simulink model "Model"  (R2020b)
settings: Solver=FixedStepDiscrete  StartTime=0.0  StopTime=inf  RelTol=1e-3
undefined symbols (not defined in the file): C12, designMultirateFIR, dt0
libraries: dspmlti4 x96, dspsrcs4 x89
(part 2 of 6)

== system Model/CORE_3_1/Path8 ==
  <IQ> : Inport
  Complex to Real-Imag : ComplexToRealImag
  Complex to Real-Imag1 : ComplexToRealImag
  Constant : Constant  Value=C12  SampleTime=dt0
  DDS_Gen1 : Subsystem
  FIR Dec1 : dspmlti4/FIR Decimation  FilterSource=Input port  h=designMultirateFIR(1,2)  D=2  filtStruct=Direct form  FilterObject=FDECIM  framing=Allow multirate processing  inputOffset=0  outputBufInitCond=0  roundingMode=Floor  overflowMode=off  firstCoeffDataTypeStr=Inherit: Same word length as input  firstCoeffMin=[]  firstCoeffMax=[]  firstCoeffLastDataTypeStr=Inherit: Same word length as input  outputDataTypeStr=Inherit: Same as accumulator  outputMin=[]  outputMax=[]  outputLastDataTypeStr=Inherit: Same as accumulator
  Freq1 : Constant  Value=2.4e6
  Mixer1 : Subsystem
  Real-Imag to Complex : RealImagToComplex
  Out1 : Outport
  wires:
  Constant/1 -> FIR Dec1/2
  Complex to Real-Imag/1 -> Mixer1/1(Input_I)
  Complex to Real-Imag1/1 -> Mixer1/3(DDS_I)
  Mixer1/2(Output_Q) -> Real-Imag to Complex/2
  Freq1/1 -> DDS_Gen1/1(In1)
  Complex to Real-Imag/2 -> Mixer1/2(Input_Q)
  Complex to Real-Imag1/2 -> Mixer1/4(DDS_Q)
  DDS_Gen1/1(Out1) -> Complex to Real-Imag1/1
  Real-Imag to Complex/1 -> FIR Dec1/1
  Mixer1/1(Output_I) -> Real-Imag to Complex/1
  FIR Dec1/1 -> Out1/1
  <IQ>/1 -> Complex to Real-Imag/1

== system Model/CORE_3_10/Path1 ==
  <IQ> : Inport
  Complex to Real-Imag : ComplexToRealImag
  Complex to Real-Imag1 : ComplexToRealImag
  Constant : Constant  Value=C12  SampleTime=dt0
  DDS_Gen1 : Subsystem
  FIR Dec1 : dspmlti4/FIR Decimation  FilterSource=Input port  h=designMultirateFIR(1,2)  D=2  filtStruct=Direct form  FilterObject=FDECIM  framing=Allow multirate processing  inputOffset=0  outputBufInitCond=0  roundingMode=Floor  overflowMode=off  firstCoeffDataTypeStr=Inherit: Same word length as input  firstCoeffMin=[]  firstCoeffMax=[]  firstCoeffLastDataTypeStr=Inherit: Same word length as input  outputDataTypeStr=Inherit: Same as accumulator  outputMin=[]  outputMax=[]  outputLastDataTypeStr=Inherit: Same as accumulator
  Freq1 : Constant  Value=2.4e6
  Mixer1 : Subsystem
  Real-Imag to Complex : RealImagToComplex
  Out1 : Outport
  wires:
  Constant/1 -> FIR Dec1/2
  Complex to Real-Imag/1 -> Mixer1/1(Input_I)
  Complex to Real-Imag1/1 -> Mixer1/3(DDS_I)
  Mixer1/2(Output_Q) -> Real-Imag to Complex/2
  Freq1/1 -> DDS_Gen1/1(In1)
  Complex to Real-Imag/2 -> Mixer1/2(Input_Q)
  Complex to Real-Imag1/2 -> Mixer1/4(DDS_Q)
  DDS_Gen1/1(Out1) -> Complex to Real-Imag1/1
  Real-Imag to Complex/1 -> FIR Dec1/1
  Mixer1/1(Output_I) -> Real-Imag to Complex/1
  FIR Dec1/1 -> Out1/1
  <IQ>/1 -> Complex to Real-Imag/1

== system Model/CORE_3_10/Path2 ==
  <IQ> : Inport
  Complex to Real-Imag : ComplexToRealImag
  Complex to Real-Imag1 : ComplexToRealImag
  Constant : Constant  Value=C12  SampleTime=dt0
  DDS_Gen1 : Subsystem
  FIR Dec1 : dspmlti4/FIR Decimation  FilterSource=Input port  h=designMultirateFIR(1,2)  D=2  filtStruct=Direct form  FilterObject=FDECIM  framing=Allow multirate processing  inputOffset=0  outputBufInitCond=0  roundingMode=Floor  overflowMode=off  firstCoeffDataTypeStr=Inherit: Same word length as input  firstCoeffMin=[]  firstCoeffMax=[]  firstCoeffLastDataTypeStr=Inherit: Same word length as input  outputDataTypeStr=Inherit: Same as accumulator  outputMin=[]  outputMax=[]  outputLastDataTypeStr=Inherit: Same as accumulator
  Freq1 : Constant  Value=2.4e6
  Mixer1 : Subsystem
  Real-Imag to Complex : RealImagToComplex
  Out1 : Outport
  wires:
  Constant/1 -> FIR Dec1/2
  Complex to Real-Imag/1 -> Mixer1/1(Input_I)
  Complex to Real-Imag1/1 -> Mixer1/3(DDS_I)
  Mixer1/2(Output_Q) -> Real-Imag to Complex/2
  Freq1/1 -> DDS_Gen1/1(In1)
  Complex to Real-Imag/2 -> Mixer1/2(Input_Q)
  Complex to Real-Imag1/2 -> Mixer1/4(DDS_Q)
  DDS_Gen1/1(Out1) -> Complex to Real-Imag1/1
  Real-Imag to Complex/1 -> FIR Dec1/1
  Mixer1/1(Output_I) -> Real-Imag to Complex/1
  FIR Dec1/1 -> Out1/1
  <IQ>/1 -> Complex to Real-Imag/1

== system Model/CORE_3_10/Path3 ==
  <IQ> : Inport
  Complex to Real-Imag : ComplexToRealImag
  Complex to Real-Imag1 : ComplexToRealImag
  Constant : Constant  Value=C12  SampleTime=dt0
  DDS_Gen1 : Subsystem
  FIR Dec1 : dspmlti4/FIR Decimation  FilterSource=Input port  h=designMultirateFIR(1,2)  D=2  filtStruct=Direct form  FilterObject=FDECIM  framing=Allow multirate processing  inputOffset=0  outputBufInitCond=0  roundingMode=Floor  overflowMode=off  firstCoeffDataTypeStr=Inherit: Same word length as input  firstCoeffMin=[]  firstCoeffMax=[]  firstCoeffLastDataTypeStr=Inherit: Same word length as input  outputDataTypeStr=Inherit: Same as accumulator  outputMin=[]  outputMax=[]  outputLastDataTypeStr=Inherit: Same as accumulator
  Freq1 : Constant  Value=2.4e6
  Mixer1 : Subsystem
  Real-Imag to Complex : RealImagToComplex
  Out1 : Outport
  wires:
  Constant/1 -> FIR Dec1/2
  Complex to Real-Imag/1 -> Mixer1/1(Input_I)
  Complex to Real-Imag1/1 -> Mixer1/3(DDS_I)
  Mixer1/2(Output_Q) -> Real-Imag to Complex/2
  Freq1/1 -> DDS_Gen1/1(In1)
  Complex to Real-Imag/2 -> Mixer1/2(Input_Q)
  Complex to Real-Imag1/2 -> Mixer1/4(DDS_Q)
  DDS_Gen1/1(Out1) -> Complex to Real-Imag1/1
  Real-Imag to Complex/1 -> FIR Dec1/1
  Mixer1/1(Output_I) -> Real-Imag to Complex/1
  FIR Dec1/1 -> Out1/1
  <IQ>/1 -> Complex to Real-Imag/1

== system Model/CORE_3_10/Path4 ==
  <IQ> : Inport
  Complex to Real-Imag : ComplexToRealImag
  Complex to Real-Imag1 : ComplexToRealImag
  Constant : Constant  Value=C12  SampleTime=dt0
  DDS_Gen1 : Subsystem
  FIR Dec1 : dspmlti4/FIR Decimation  FilterSource=Input port  h=designMultirateFIR(1,2)  D=2  filtStruct=Direct form  FilterObject=FDECIM  framing=Allow multirate processing  inputOffset=0  outputBufInitCond=0  roundingMode=Floor  overflowMode=off  firstCoeffDataTypeStr=Inherit: Same word length as input  firstCoeffMin=[]  firstCoeffMax=[]  firstCoeffLastDataTypeStr=Inherit: Same word length as input  outputDataTypeStr=Inherit: Same as accumulator  outputMin=[]  outputMax=[]  outputLastDataTypeStr=Inherit: Same as accumulator
  Freq1 : Constant  Value=2.4e6
  Mixer1 : Subsystem
  Real-Imag to Complex : RealImagToComplex
  Out1 : Outport
  wires:
  Constant/1 -> FIR Dec1/2
  Complex to Real-Imag/1 -> Mixer1/1(Input_I)
  Complex to Real-Imag1/1 -> Mixer1/3(DDS_I)
  Mixer1/2(Output_Q) -> Real-Imag to Complex/2
  Freq1/1 -> DDS_Gen1/1(In1)
  Complex to Real-Imag/2 -> Mixer1/2(Input_Q)
  Complex to Real-Imag1/2 -> Mixer1/4(DDS_Q)
  DDS_Gen1/1(Out1) -> Complex to Real-Imag1/1
  Real-Imag to Complex/1 -> FIR Dec1/1
  Mixer1/1(Output_I) -> Real-Imag to Complex/1
  FIR Dec1/1 -> Out1/1
  <IQ>/1 -> Complex to Real-Imag/1

== system Model/CORE_3_10/Path5 ==
  <IQ> : Inport
  Complex to Real-Imag : ComplexToRealImag
  Complex to Real-Imag1 : ComplexToRealImag
  Constant : Constant  Value=C12  SampleTime=dt0
  DDS_Gen1 : Subsystem
  FIR Dec1 : dspmlti4/FIR Decimation  FilterSource=Input port  h=designMultirateFIR(1,2)  D=2  filtStruct=Direct form  FilterObject=FDECIM  framing=Allow multirate processing  inputOffset=0  outputBufInitCond=0  roundingMode=Floor  overflowMode=off  firstCoeffDataTypeStr=Inherit: Same word length as input  firstCoeffMin=[]  firstCoeffMax=[]  firstCoeffLastDataTypeStr=Inherit: Same word length as input  outputDataTypeStr=Inherit: Same as accumulator  outputMin=[]  outputMax=[]  outputLastDataTypeStr=Inherit: Same as accumulator
  Freq1 : Constant  Value=2.4e6
  Mixer1 : Subsystem
  Real-Imag to Complex : RealImagToComplex
  Out1 : Outport
  wires:
  Constant/1 -> FIR Dec1/2
  Complex to Real-Imag/1 -> Mixer1/1(Input_I)
  Complex to Real-Imag1/1 -> Mixer1/3(DDS_I)
  Mixer1/2(Output_Q) -> Real-Imag to Complex/2
  Freq1/1 -> DDS_Gen1/1(In1)
  Complex to Real-Imag/2 -> Mixer1/2(Input_Q)
  Complex to Real-Imag1/2 -> Mixer1/4(DDS_Q)
  DDS_Gen1/1(Out1) -> Complex to Real-Imag1/1
  Real-Imag to Complex/1 -> FIR Dec1/1
  Mixer1/1(Output_I) -> Real-Imag to Complex/1
  FIR Dec1/1 -> Out1/1
  <IQ>/1 -> Complex to Real-Imag/1

== system Model/CORE_3_10/Path6 ==
  <IQ> : Inport
  Complex to Real-Imag : ComplexToRealImag
  Complex to Real-Imag1 : ComplexToRealImag
  Constant : Constant  Value=C12  SampleTime=dt0
  DDS_Gen1 : Subsystem
  FIR Dec1 : dspmlti4/FIR Decimation  FilterSource=Input port  h=designMultirateFIR(1,2)  D=2  filtStruct=Direct form  FilterObject=FDECIM  framing=Allow multirate processing  inputOffset=0  outputBufInitCond=0  roundingMode=Floor  overflowMode=off  firstCoeffDataTypeStr=Inherit: Same word length as input  firstCoeffMin=[]  firstCoeffMax=[]  firstCoeffLastDataTypeStr=Inherit: Same word length as input  outputDataTypeStr=Inherit: Same as accumulator  outputMin=[]  outputMax=[]  outputLastDataTypeStr=Inherit: Same as accumulator
  Freq1 : Constant  Value=2.4e6
  Mixer1 : Subsystem
  Real-Imag to Complex : RealImagToComplex
  Out1 : Outport
  wires:
  Constant/1 -> FIR Dec1/2
  Complex to Real-Imag/1 -> Mixer1/1(Input_I)
  Complex to Real-Imag1/1 -> Mixer1/3(DDS_I)
  Mixer1/2(Output_Q) -> Real-Imag to Complex/2
  Freq1/1 -> DDS_Gen1/1(In1)
  Complex to Real-Imag/2 -> Mixer1/2(Input_Q)
  Complex to Real-Imag1/2 -> Mixer1/4(DDS_Q)
  DDS_Gen1/1(Out1) -> Complex to Real-Imag1/1
  Real-Imag to Complex/1 -> FIR Dec1/1
  Mixer1/1(Output_I) -> Real-Imag to Complex/1
  FIR Dec1/1 -> Out1/1
  <IQ>/1 -> Complex to Real-Imag/1

== system Model/CORE_3_10/Path7 ==
  <IQ> : Inport
  Complex to Real-Imag : ComplexToRealImag
  Complex to Real-Imag1 : ComplexToRealImag
  Constant : Constant  Value=C12  SampleTime=dt0
  DDS_Gen1 : Subsystem
  FIR Dec1 : dspmlti4/FIR Decimation  FilterSource=Input port  h=designMultirateFIR(1,2)  D=2  filtStruct=Direct form  FilterObject=FDECIM  framing=Allow multirate processing  inputOffset=0  outputBufInitCond=0  roundingMode=Floor  overflowMode=off  firstCoeffDataTypeStr=Inherit: Same word length as input  firstCoeffMin=[]  firstCoeffMax=[]  firstCoeffLastDataTypeStr=Inherit: Same word length as input  outputDataTypeStr=Inherit: Same as accumulator  outputMin=[]  outputMax=[]  outputLastDataTypeStr=Inherit: Same as accumulator
  Freq1 : Constant  Value=2.4e6
  Mixer1 : Subsystem
  Real-Imag to Complex : RealImagToComplex
  Out1 : Outport
  wires:
  Constant/1 -> FIR Dec1/2
  Complex to Real-Imag/1 -> Mixer1/1(Input_I)
  Complex to Real-Imag1/1 -> Mixer1/3(DDS_I)
  Mixer1/2(Output_Q) -> Real-Imag to Complex/2
  Freq1/1 -> DDS_Gen1/1(In1)
  Complex to Real-Imag/2 -> Mixer1/2(Input_Q)
  Complex to Real-Imag1/2 -> Mixer1/4(DDS_Q)
  DDS_Gen1/1(Out1) -> Complex to Real-Imag1/1
  Real-Imag to Complex/1 -> FIR Dec1/1
  Mixer1/1(Output_I) -> Real-Imag to Complex/1
  FIR Dec1/1 -> Out1/1
  <IQ>/1 -> Complex to Real-Imag/1

== system Model/CORE_3_10/Path8 ==
  <IQ> : Inport
  Complex to Real-Imag : ComplexToRealImag
  Complex to Real-Imag1 : ComplexToRealImag
  Constant : Constant  Value=C12  SampleTime=dt0
  DDS_Gen1 : Subsystem
  FIR Dec1 : dspmlti4/FIR Decimation  FilterSource=Input port  h=designMultirateFIR(1,2)  D=2  filtStruct=Direct form  FilterObject=FDECIM  framing=Allow multirate processing  inputOffset=0  outputBufInitCond=0  roundingMode=Floor  overflowMode=off  firstCoeffDataTypeStr=Inherit: Same word length as input  firstCoeffMin=[]  firstCoeffMax=[]  firstCoeffLastDataTypeStr=Inherit: Same word length as input  outputDataTypeStr=Inherit: Same as accumulator  outputMin=[]  outputMax=[]  outputLastDataTypeStr=Inherit: Same as accumulator
  Freq1 : Constant  Value=2.4e6
  Mixer1 : Subsystem
  Real-Imag to Complex : RealImagToComplex
  Out1 : Outport
  wires:
  Constant/1 -> FIR Dec1/2
  Complex to Real-Imag/1 -> Mixer1/1(Input_I)
  Complex to Real-Imag1/1 -> Mixer1/3(DDS_I)
  Mixer1/2(Output_Q) -> Real-Imag to Complex/2
  Freq1/1 -> DDS_Gen1/1(In1)
  Complex to Real-Imag/2 -> Mixer1/2(Input_Q)
  Complex to Real-Imag1/2 -> Mixer1/4(DDS_Q)
  DDS_Gen1/1(Out1) -> Complex to Real-Imag1/1
  Real-Imag to Complex/1 -> FIR Dec1/1
  Mixer1/1(Output_I) -> Real-Imag to Complex/1
  FIR Dec1/1 -> Out1/1
  <IQ>/1 -> Complex to Real-Imag/1

== system Model/CORE_3_2/Path1 ==
  <IQ> : Inport
  Complex to Real-Imag : ComplexToRealImag
  Complex to Real-Imag1 : ComplexToRealImag
  Constant : Constant  Value=C12  SampleTime=dt0
  DDS_Gen1 : Subsystem
  FIR Dec1 : dspmlti4/FIR Decimation  FilterSource=Input port  h=designMultirateFIR(1,2)  D=2  filtStruct=Direct form  FilterObject=FDECIM  framing=Allow multirate processing  inputOffset=0  outputBufInitCond=0  roundingMode=Floor  overflowMode=off  firstCoeffDataTypeStr=Inherit: Same word length as input  firstCoeffMin=[]  firstCoeffMax=[]  firstCoeffLastDataTypeStr=Inherit: Same word length as input  outputDataTypeStr=Inherit: Same as accumulator  outputMin=[]  outputMax=[]  outputLastDataTypeStr=Inherit: Same as accumulator
  Freq1 : Constant  Value=2.4e6
  Mixer1 : Subsystem
  Real-Imag to Complex : RealImagToComplex
  Out1 : Outport
  wires:
  Constant/1 -> FIR Dec1/2
  Complex to Real-Imag/1 -> Mixer1/1(Input_I)
  Complex to Real-Imag1/1 -> Mixer1/3(DDS_I)
  Mixer1/2(Output_Q) -> Real-Imag to Complex/2
  Freq1/1 -> DDS_Gen1/1(In1)
  Complex to Real-Imag/2 -> Mixer1/2(Input_Q)
  Complex to Real-Imag1/2 -> Mixer1/4(DDS_Q)
  DDS_Gen1/1(Out1) -> Complex to Real-Imag1/1
  Real-Imag to Complex/1 -> FIR Dec1/1
  Mixer1/1(Output_I) -> Real-Imag to Complex/1
  FIR Dec1/1 -> Out1/1
  <IQ>/1 -> Complex to Real-Imag/1

== system Model/CORE_3_2/Path2 ==
  <IQ> : Inport
  Complex to Real-Imag : ComplexToRealImag
  Complex to Real-Imag1 : ComplexToRealImag
  Constant : Constant  Value=C12  SampleTime=dt0
  DDS_Gen1 : Subsystem
  FIR Dec1 : dspmlti4/FIR Decimation  FilterSource=Input port  h=designMultirateFIR(1,2)  D=2  filtStruct=Direct form  FilterObject=FDECIM  framing=Allow multirate processing  inputOffset=0  outputBufInitCond=0  roundingMode=Floor  overflowMode=off  firstCoeffDataTypeStr=Inherit: Same word length as input  firstCoeffMin=[]  firstCoeffMax=[]  firstCoeffLastDataTypeStr=Inherit: Same word length as input  outputDataTypeStr=Inherit: Same as accumulator  outputMin=[]  outputMax=[]  outputLastDataTypeStr=Inherit: Same as accumulator
  Freq1 : Constant  Value=2.4e6
  Mixer1 : Subsystem
  Real-Imag to Complex : RealImagToComplex
  Out1 : Outport
  wires:
  Constant/1 -> FIR Dec1/2
  Complex to Real-Imag/1 -> Mixer1/1(Input_I)
  Complex to Real-Imag1/1 -> Mixer1/3(DDS_I)
  Mixer1/2(Output_Q) -> Real-Imag to Complex/2
  Freq1/1 -> DDS_Gen1/1(In1)
  Complex to Real-Imag/2 -> Mixer1/2(Input_Q)
  Complex to Real-Imag1/2 -> Mixer1/4(DDS_Q)
  DDS_Gen1/1(Out1) -> Complex to Real-Imag1/1
  Real-Imag to Complex/1 -> FIR Dec1/1
  Mixer1/1(Output_I) -> Real-Imag to Complex/1
  FIR Dec1/1 -> Out1/1
  <IQ>/1 -> Complex to Real-Imag/1

== system Model/CORE_3_2/Path3 ==
  <IQ> : Inport
  Complex to Real-Imag : ComplexToRealImag
  Complex to Real-Imag1 : ComplexToRealImag
  Constant : Constant  Value=C12  SampleTime=dt0
  DDS_Gen1 : Subsystem
  FIR Dec1 : dspmlti4/FIR Decimation  FilterSource=Input port  h=designMultirateFIR(1,2)  D=2  filtStruct=Direct form  FilterObject=FDECIM  framing=Allow multirate processing  inputOffset=0  outputBufInitCond=0  roundingMode=Floor  overflowMode=off  firstCoeffDataTypeStr=Inherit: Same word length as input  firstCoeffMin=[]  firstCoeffMax=[]  firstCoeffLastDataTypeStr=Inherit: Same word length as input  outputDataTypeStr=Inherit: Same as accumulator  outputMin=[]  outputMax=[]  outputLastDataTypeStr=Inherit: Same as accumulator
  Freq1 : Constant  Value=2.4e6
  Mixer1 : Subsystem
  Real-Imag to Complex : RealImagToComplex
  Out1 : Outport
  wires:
  Constant/1 -> FIR Dec1/2
  Complex to Real-Imag/1 -> Mixer1/1(Input_I)
  Complex to Real-Imag1/1 -> Mixer1/3(DDS_I)
  Mixer1/2(Output_Q) -> Real-Imag to Complex/2
  Freq1/1 -> DDS_Gen1/1(In1)
  Complex to Real-Imag/2 -> Mixer1/2(Input_Q)
  Complex to Real-Imag1/2 -> Mixer1/4(DDS_Q)
  DDS_Gen1/1(Out1) -> Complex to Real-Imag1/1
  Real-Imag to Complex/1 -> FIR Dec1/1
  Mixer1/1(Output_I) -> Real-Imag to Complex/1
  FIR Dec1/1 -> Out1/1
  <IQ>/1 -> Complex to Real-Imag/1

== system Model/CORE_3_2/Path4 ==
  <IQ> : Inport
  Complex to Real-Imag : ComplexToRealImag
  Complex to Real-Imag1 : ComplexToRealImag
  Constant : Constant  Value=C12  SampleTime=dt0
  DDS_Gen1 : Subsystem
  FIR Dec1 : dspmlti4/FIR Decimation  FilterSource=Input port  h=designMultirateFIR(1,2)  D=2  filtStruct=Direct form  FilterObject=FDECIM  framing=Allow multirate processing  inputOffset=0  outputBufInitCond=0  roundingMode=Floor  overflowMode=off  firstCoeffDataTypeStr=Inherit: Same word length as input  firstCoeffMin=[]  firstCoeffMax=[]  firstCoeffLastDataTypeStr=Inherit: Same word length as input  outputDataTypeStr=Inherit: Same as accumulator  outputMin=[]  outputMax=[]  outputLastDataTypeStr=Inherit: Same as accumulator
  Freq1 : Constant  Value=2.4e6
  Mixer1 : Subsystem
  Real-Imag to Complex : RealImagToComplex
  Out1 : Outport
  wires:
  Constant/1 -> FIR Dec1/2
  Complex to Real-Imag/1 -> Mixer1/1(Input_I)
  Complex to Real-Imag1/1 -> Mixer1/3(DDS_I)
  Mixer1/2(Output_Q) -> Real-Imag to Complex/2
  Freq1/1 -> DDS_Gen1/1(In1)
  Complex to Real-Imag/2 -> Mixer1/2(Input_Q)
  Complex to Real-Imag1/2 -> Mixer1/4(DDS_Q)
  DDS_Gen1/1(Out1) -> Complex to Real-Imag1/1
  Real-Imag to Complex/1 -> FIR Dec1/1
  Mixer1/1(Output_I) -> Real-Imag to Complex/1
  FIR Dec1/1 -> Out1/1
  <IQ>/1 -> Complex to Real-Imag/1

== system Model/CORE_3_2/Path5 ==
  <IQ> : Inport
  Complex to Real-Imag : ComplexToRealImag
  Complex to Real-Imag1 : ComplexToRealImag
  Constant : Constant  Value=C12  SampleTime=dt0
  DDS_Gen1 : Subsystem
  FIR Dec1 : dspmlti4/FIR Decimation  FilterSource=Input port  h=designMultirateFIR(1,2)  D=2  filtStruct=Direct form  FilterObject=FDECIM  framing=Allow multirate processing  inputOffset=0  outputBufInitCond=0  roundingMode=Floor  overflowMode=off  firstCoeffDataTypeStr=Inherit: Same word length as input  firstCoeffMin=[]  firstCoeffMax=[]  firstCoeffLastDataTypeStr=Inherit: Same word length as input  outputDataTypeStr=Inherit: Same as accumulator  outputMin=[]  outputMax=[]  outputLastDataTypeStr=Inherit: Same as accumulator
  Freq1 : Constant  Value=2.4e6
  Mixer1 : Subsystem
  Real-Imag to Complex : RealImagToComplex
  Out1 : Outport
  wires:
  Constant/1 -> FIR Dec1/2
  Complex to Real-Imag/1 -> Mixer1/1(Input_I)
  Complex to Real-Imag1/1 -> Mixer1/3(DDS_I)
  Mixer1/2(Output_Q) -> Real-Imag to Complex/2
  Freq1/1 -> DDS_Gen1/1(In1)
  Complex to Real-Imag/2 -> Mixer1/2(Input_Q)
  Complex to Real-Imag1/2 -> Mixer1/4(DDS_Q)
  DDS_Gen1/1(Out1) -> Complex to Real-Imag1/1
  Real-Imag to Complex/1 -> FIR Dec1/1
  Mixer1/1(Output_I) -> Real-Imag to Complex/1
  FIR Dec1/1 -> Out1/1
  <IQ>/1 -> Complex to Real-Imag/1

== system Model/CORE_3_2/Path6 ==
  <IQ> : Inport
  Complex to Real-Imag : ComplexToRealImag
  Complex to Real-Imag1 : ComplexToRealImag
  Constant : Constant  Value=C12  SampleTime=dt0
  DDS_Gen1 : Subsystem
  FIR Dec1 : dspmlti4/FIR Decimation  FilterSource=Input port  h=designMultirateFIR(1,2)  D=2  filtStruct=Direct form  FilterObject=FDECIM  framing=Allow multirate processing  inputOffset=0  outputBufInitCond=0  roundingMode=Floor  overflowMode=off  firstCoeffDataTypeStr=Inherit: Same word length as input  firstCoeffMin=[]  firstCoeffMax=[]  firstCoeffLastDataTypeStr=Inherit: Same word length as input  outputDataTypeStr=Inherit: Same as accumulator  outputMin=[]  outputMax=[]  outputLastDataTypeStr=Inherit: Same as accumulator
  Freq1 : Constant  Value=2.4e6
  Mixer1 : Subsystem
  Real-Imag to Complex : RealImagToComplex
  Out1 : Outport
  wires:
  Constant/1 -> FIR Dec1/2
  Complex to Real-Imag/1 -> Mixer1/1(Input_I)
  Complex to Real-Imag1/1 -> Mixer1/3(DDS_I)
  Mixer1/2(Output_Q) -> Real-Imag to Complex/2
  Freq1/1 -> DDS_Gen1/1(In1)
  Complex to Real-Imag/2 -> Mixer1/2(Input_Q)
  Complex to Real-Imag1/2 -> Mixer1/4(DDS_Q)
  DDS_Gen1/1(Out1) -> Complex to Real-Imag1/1
  Real-Imag to Complex/1 -> FIR Dec1/1
  Mixer1/1(Output_I) -> Real-Imag to Complex/1
  FIR Dec1/1 -> Out1/1
  <IQ>/1 -> Complex to Real-Imag/1

== system Model/CORE_3_2/Path7 ==
  <IQ> : Inport
  Complex to Real-Imag : ComplexToRealImag
  Complex to Real-Imag1 : ComplexToRealImag
  Constant : Constant  Value=C12  SampleTime=dt0
  DDS_Gen1 : Subsystem
  FIR Dec1 : dspmlti4/FIR Decimation  FilterSource=Input port  h=designMultirateFIR(1,2)  D=2  filtStruct=Direct form  FilterObject=FDECIM  framing=Allow multirate processing  inputOffset=0  outputBufInitCond=0  roundingMode=Floor  overflowMode=off  firstCoeffDataTypeStr=Inherit: Same word length as input  firstCoeffMin=[]  firstCoeffMax=[]  firstCoeffLastDataTypeStr=Inherit: Same word length as input  outputDataTypeStr=Inherit: Same as accumulator  outputMin=[]  outputMax=[]  outputLastDataTypeStr=Inherit: Same as accumulator
  Freq1 : Constant  Value=2.4e6
  Mixer1 : Subsystem
  Real-Imag to Complex : RealImagToComplex
  Out1 : Outport
  wires:
  Constant/1 -> FIR Dec1/2
  Complex to Real-Imag/1 -> Mixer1/1(Input_I)
  Complex to Real-Imag1/1 -> Mixer1/3(DDS_I)
  Mixer1/2(Output_Q) -> Real-Imag to Complex/2
  Freq1/1 -> DDS_Gen1/1(In1)
  Complex to Real-Imag/2 -> Mixer1/2(Input_Q)
  Complex to Real-Imag1/2 -> Mixer1/4(DDS_Q)
  DDS_Gen1/1(Out1) -> Complex to Real-Imag1/1
  Real-Imag to Complex/1 -> FIR Dec1/1
  Mixer1/1(Output_I) -> Real-Imag to Complex/1
  FIR Dec1/1 -> Out1/1
  <IQ>/1 -> Complex to Real-Imag/1

== system Model/CORE_3_2/Path8 ==
  <IQ> : Inport
  Complex to Real-Imag : ComplexToRealImag
  Complex to Real-Imag1 : ComplexToRealImag
  Constant : Constant  Value=C12  SampleTime=dt0
  DDS_Gen1 : Subsystem
  FIR Dec1 : dspmlti4/FIR Decimation  FilterSource=Input port  h=designMultirateFIR(1,2)  D=2  filtStruct=Direct form  FilterObject=FDECIM  framing=Allow multirate processing  inputOffset=0  outputBufInitCond=0  roundingMode=Floor  overflowMode=off  firstCoeffDataTypeStr=Inherit: Same word length as input  firstCoeffMin=[]  firstCoeffMax=[]  firstCoeffLastDataTypeStr=Inherit: Same word length as input  outputDataTypeStr=Inherit: Same as accumulator  outputMin=[]  outputMax=[]  outputLastDataTypeStr=Inherit: Same as accumulator
  Freq1 : Constant  Value=2.4e6
  Mixer1 : Subsystem
  Real-Imag to Complex : RealImagToComplex
  Out1 : Outport
  wires:
  Constant/1 -> FIR Dec1/2
  Complex to Real-Imag/1 -> Mixer1/1(Input_I)
  Complex to Real-Imag1/1 -> Mixer1/3(DDS_I)
  Mixer1/2(Output_Q) -> Real-Imag to Complex/2
  Freq1/1 -> DDS_Gen1/1(In1)
  Complex to Real-Imag/2 -> Mixer1/2(Input_Q)
  Complex to Real-Imag1/2 -> Mixer1/4(DDS_Q)
  DDS_Gen1/1(Out1) -> Complex to Real-Imag1/1
  Real-Imag to Complex/1 -> FIR Dec1/1
  Mixer1/1(Output_I) -> Real-Imag to Complex/1
  FIR Dec1/1 -> Out1/1
  <IQ>/1 -> Complex to Real-Imag/1

== system Model/CORE_3_3/Path1 ==
  <IQ> : Inport
  Complex to Real-Imag : ComplexToRealImag
  Complex to Real-Imag1 : ComplexToRealImag
  Constant : Constant  Value=C12  SampleTime=dt0
  DDS_Gen1 : Subsystem
  FIR Dec1 : dspmlti4/FIR Decimation  FilterSource=Input port  h=designMultirateFIR(1,2)  D=2  filtStruct=Direct form  FilterObject=FDECIM  framing=Allow multirate processing  inputOffset=0  outputBufInitCond=0  roundingMode=Floor  overflowMode=off  firstCoeffDataTypeStr=Inherit: Same word length as input  firstCoeffMin=[]  firstCoeffMax=[]  firstCoeffLastDataTypeStr=Inherit: Same word length as input  outputDataTypeStr=Inherit: Same as accumulator  outputMin=[]  outputMax=[]  outputLastDataTypeStr=Inherit: Same as accumulator
  Freq1 : Constant  Value=2.4e6
  Mixer1 : Subsystem
  Real-Imag to Complex : RealImagToComplex
  Out1 : Outport
  wires:
  Constant/1 -> FIR Dec1/2
  Complex to Real-Imag/1 -> Mixer1/1(Input_I)
  Complex to Real-Imag1/1 -> Mixer1/3(DDS_I)
  Mixer1/2(Output_Q) -> Real-Imag to Complex/2
  Freq1/1 -> DDS_Gen1/1(In1)
  Complex to Real-Imag/2 -> Mixer1/2(Input_Q)
  Complex to Real-Imag1/2 -> Mixer1/4(DDS_Q)
  DDS_Gen1/1(Out1) -> Complex to Real-Imag1/1
  Real-Imag to Complex/1 -> FIR Dec1/1
  Mixer1/1(Output_I) -> Real-Imag to Complex/1
  FIR Dec1/1 -> Out1/1
  <IQ>/1 -> Complex to Real-Imag/1

== system Model/CORE_3_3/Path2 ==
  <IQ> : Inport
  Complex to Real-Imag : ComplexToRealImag
  Complex to Real-Imag1 : ComplexToRealImag
  Constant : Constant  Value=C12  SampleTime=dt0
  DDS_Gen1 : Subsystem
  FIR Dec1 : dspmlti4/FIR Decimation  FilterSource=Input port  h=designMultirateFIR(1,2)  D=2  filtStruct=Direct form  FilterObject=FDECIM  framing=Allow multirate processing  inputOffset=0  outputBufInitCond=0  roundingMode=Floor  overflowMode=off  firstCoeffDataTypeStr=Inherit: Same word length as input  firstCoeffMin=[]  firstCoeffMax=[]  firstCoeffLastDataTypeStr=Inherit: Same word length as input  outputDataTypeStr=Inherit: Same as accumulator  outputMin=[]  outputMax=[]  outputLastDataTypeStr=Inherit: Same as accumulator
  Freq1 : Constant  Value=2.4e6
  Mixer1 : Subsystem
  Real-Imag to Complex : RealImagToComplex
  Out1 : Outport
  wires:
  Constant/1 -> FIR Dec1/2
  Complex to Real-Imag/1 -> Mixer1/1(Input_I)
  Complex to Real-Imag1/1 -> Mixer1/3(DDS_I)
  Mixer1/2(Output_Q) -> Real-Imag to Complex/2
  Freq1/1 -> DDS_Gen1/1(In1)
  Complex to Real-Imag/2 -> Mixer1/2(Input_Q)
  Complex to Real-Imag1/2 -> Mixer1/4(DDS_Q)
  DDS_Gen1/1(Out1) -> Complex to Real-Imag1/1
  Real-Imag to Complex/1 -> FIR Dec1/1
  Mixer1/1(Output_I) -> Real-Imag to Complex/1
  FIR Dec1/1 -> Out1/1
  <IQ>/1 -> Complex to Real-Imag/1

== system Model/CORE_3_3/Path3 ==
  <IQ> : Inport
  Complex to Real-Imag : ComplexToRealImag
  Complex to Real-Imag1 : ComplexToRealImag
  Constant : Constant  Value=C12  SampleTime=dt0
  DDS_Gen1 : Subsystem
  FIR Dec1 : dspmlti4/FIR Decimation  FilterSource=Input port  h=designMultirateFIR(1,2)  D=2  filtStruct=Direct form  FilterObject=FDECIM  framing=Allow multirate processing  inputOffset=0  outputBufInitCond=0  roundingMode=Floor  overflowMode=off  firstCoeffDataTypeStr=Inherit: Same word length as input  firstCoeffMin=[]  firstCoeffMax=[]  firstCoeffLastDataTypeStr=Inherit: Same word length as input  outputDataTypeStr=Inherit: Same as accumulator  outputMin=[]  outputMax=[]  outputLastDataTypeStr=Inherit: Same as accumulator
  Freq1 : Constant  Value=2.4e6
  Mixer1 : Subsystem
  Real-Imag to Complex : RealImagToComplex
  Out1 : Outport
  wires:
  Constant/1 -> FIR Dec1/2
  Complex to Real-Imag/1 -> Mixer1/1(Input_I)
  Complex to Real-Imag1/1 -> Mixer1/3(DDS_I)
  Mixer1/2(Output_Q) -> Real-Imag to Complex/2
  Freq1/1 -> DDS_Gen1/1(In1)
  Complex to Real-Imag/2 -> Mixer1/2(Input_Q)
  Complex to Real-Imag1/2 -> Mixer1/4(DDS_Q)
  DDS_Gen1/1(Out1) -> Complex to Real-Imag1/1
  Real-Imag to Complex/1 -> FIR Dec1/1
  Mixer1/1(Output_I) -> Real-Imag to Complex/1
  FIR Dec1/1 -> Out1/1
  <IQ>/1 -> Complex to Real-Imag/1

== system Model/CORE_3_3/Path4 ==
  <IQ> : Inport
  Complex to Real-Imag : ComplexToRealImag
  Complex to Real-Imag1 : ComplexToRealImag
  Constant : Constant  Value=C12  SampleTime=dt0
  DDS_Gen1 : Subsystem
  FIR Dec1 : dspmlti4/FIR Decimation  FilterSource=Input port  h=designMultirateFIR(1,2)  D=2  filtStruct=Direct form  FilterObject=FDECIM  framing=Allow multirate processing  inputOffset=0  outputBufInitCond=0  roundingMode=Floor  overflowMode=off  firstCoeffDataTypeStr=Inherit: Same word length as input  firstCoeffMin=[]  firstCoeffMax=[]  firstCoeffLastDataTypeStr=Inherit: Same word length as input  outputDataTypeStr=Inherit: Same as accumulator  outputMin=[]  outputMax=[]  outputLastDataTypeStr=Inherit: Same as accumulator
  Freq1 : Constant  Value=2.4e6
  Mixer1 : Subsystem
  Real-Imag to Complex : RealImagToComplex
  Out1 : Outport
  wires:
  Constant/1 -> FIR Dec1/2
  Complex to Real-Imag/1 -> Mixer1/1(Input_I)
  Complex to Real-Imag1/1 -> Mixer1/3(DDS_I)
  Mixer1/2(Output_Q) -> Real-Imag to Complex/2
  Freq1/1 -> DDS_Gen1/1(In1)
  Complex to Real-Imag/2 -> Mixer1/2(Input_Q)
  Complex to Real-Imag1/2 -> Mixer1/4(DDS_Q)
  DDS_Gen1/1(Out1) -> Complex to Real-Imag1/1
  Real-Imag to Complex/1 -> FIR Dec1/1
  Mixer1/1(Output_I) -> Real-Imag to Complex/1
  FIR Dec1/1 -> Out1/1
  <IQ>/1 -> Complex to Real-Imag/1

== system Model/CORE_3_3/Path5 ==
  <IQ> : Inport
  Complex to Real-Imag : ComplexToRealImag
  Complex to Real-Imag1 : ComplexToRealImag
  Constant : Constant  Value=C12  SampleTime=dt0
  DDS_Gen1 : Subsystem
  FIR Dec1 : dspmlti4/FIR Decimation  FilterSource=Input port  h=designMultirateFIR(1,2)  D=2  filtStruct=Direct form  FilterObject=FDECIM  framing=Allow multirate processing  inputOffset=0  outputBufInitCond=0  roundingMode=Floor  overflowMode=off  firstCoeffDataTypeStr=Inherit: Same word length as input  firstCoeffMin=[]  firstCoeffMax=[]  firstCoeffLastDataTypeStr=Inherit: Same word length as input  outputDataTypeStr=Inherit: Same as accumulator  outputMin=[]  outputMax=[]  outputLastDataTypeStr=Inherit: Same as accumulator
  Freq1 : Constant  Value=2.4e6
  Mixer1 : Subsystem
  Real-Imag to Complex : RealImagToComplex
  Out1 : Outport
  wires:
  Constant/1 -> FIR Dec1/2
  Complex to Real-Imag/1 -> Mixer1/1(Input_I)
  Complex to Real-Imag1/1 -> Mixer1/3(DDS_I)
  Mixer1/2(Output_Q) -> Real-Imag to Complex/2
  Freq1/1 -> DDS_Gen1/1(In1)
  Complex to Real-Imag/2 -> Mixer1/2(Input_Q)
  Complex to Real-Imag1/2 -> Mixer1/4(DDS_Q)
  DDS_Gen1/1(Out1) -> Complex to Real-Imag1/1
  Real-Imag to Complex/1 -> FIR Dec1/1
  Mixer1/1(Output_I) -> Real-Imag to Complex/1
  FIR Dec1/1 -> Out1/1
  <IQ>/1 -> Complex to Real-Imag/1

== system Model/CORE_3_3/Path6 ==
  <IQ> : Inport
  Complex to Real-Imag : ComplexToRealImag
  Complex to Real-Imag1 : ComplexToRealImag
  Constant : Constant  Value=C12  SampleTime=dt0
  DDS_Gen1 : Subsystem
  FIR Dec1 : dspmlti4/FIR Decimation  FilterSource=Input port  h=designMultirateFIR(1,2)  D=2  filtStruct=Direct form  FilterObject=FDECIM  framing=Allow multirate processing  inputOffset=0  outputBufInitCond=0  roundingMode=Floor  overflowMode=off  firstCoeffDataTypeStr=Inherit: Same word length as input  firstCoeffMin=[]  firstCoeffMax=[]  firstCoeffLastDataTypeStr=Inherit: Same word length as input  outputDataTypeStr=Inherit: Same as accumulator  outputMin=[]  outputMax=[]  outputLastDataTypeStr=Inherit: Same as accumulator
  Freq1 : Constant  Value=2.4e6
  Mixer1 : Subsystem
  Real-Imag to Complex : RealImagToComplex
  Out1 : Outport
  wires:
  Constant/1 -> FIR Dec1/2
  Complex to Real-Imag/1 -> Mixer1/1(Input_I)
  Complex to Real-Imag1/1 -> Mixer1/3(DDS_I)
  Mixer1/2(Output_Q) -> Real-Imag to Complex/2
  Freq1/1 -> DDS_Gen1/1(In1)
  Complex to Real-Imag/2 -> Mixer1/2(Input_Q)
  Complex to Real-Imag1/2 -> Mixer1/4(DDS_Q)
  DDS_Gen1/1(Out1) -> Complex to Real-Imag1/1
  Real-Imag to Complex/1 -> FIR Dec1/1
  Mixer1/1(Output_I) -> Real-Imag to Complex/1
  FIR Dec1/1 -> Out1/1
  <IQ>/1 -> Complex to Real-Imag/1

== system Model/CORE_3_3/Path7 ==
  <IQ> : Inport
  Complex to Real-Imag : ComplexToRealImag
  Complex to Real-Imag1 : ComplexToRealImag
  Constant : Constant  Value=C12  SampleTime=dt0
  DDS_Gen1 : Subsystem
  FIR Dec1 : dspmlti4/FIR Decimation  FilterSource=Input port  h=designMultirateFIR(1,2)  D=2  filtStruct=Direct form  FilterObject=FDECIM  framing=Allow multirate processing  inputOffset=0  outputBufInitCond=0  roundingMode=Floor  overflowMode=off  firstCoeffDataTypeStr=Inherit: Same word length as input  firstCoeffMin=[]  firstCoeffMax=[]  firstCoeffLastDataTypeStr=Inherit: Same word length as input  outputDataTypeStr=Inherit: Same as accumulator  outputMin=[]  outputMax=[]  outputLastDataTypeStr=Inherit: Same as accumulator
  Freq1 : Constant  Value=2.4e6
  Mixer1 : Subsystem
  Real-Imag to Complex : RealImagToComplex
  Out1 : Outport
  wires:
  Constant/1 -> FIR Dec1/2
  Complex to Real-Imag/1 -> Mixer1/1(Input_I)
  Complex to Real-Imag1/1 -> Mixer1/3(DDS_I)
  Mixer1/2(Output_Q) -> Real-Imag to Complex/2
  Freq1/1 -> DDS_Gen1/1(In1)
  Complex to Real-Imag/2 -> Mixer1/2(Input_Q)
  Complex to Real-Imag1/2 -> Mixer1/4(DDS_Q)
  DDS_Gen1/1(Out1) -> Complex to Real-Imag1/1
  Real-Imag to Complex/1 -> FIR Dec1/1
  Mixer1/1(Output_I) -> Real-Imag to Complex/1
  FIR Dec1/1 -> Out1/1
  <IQ>/1 -> Complex to Real-Imag/1

== system Model/CORE_3_3/Path8 ==
  <IQ> : Inport
  Complex to Real-Imag : ComplexToRealImag
  Complex to Real-Imag1 : ComplexToRealImag
  Constant : Constant  Value=C12  SampleTime=dt0
  DDS_Gen1 : Subsystem
  FIR Dec1 : dspmlti4/FIR Decimation  FilterSource=Input port  h=designMultirateFIR(1,2)  D=2  filtStruct=Direct form  FilterObject=FDECIM  framing=Allow multirate processing  inputOffset=0  outputBufInitCond=0  roundingMode=Floor  overflowMode=off  firstCoeffDataTypeStr=Inherit: Same word length as input  firstCoeffMin=[]  firstCoeffMax=[]  firstCoeffLastDataTypeStr=Inherit: Same word length as input  outputDataTypeStr=Inherit: Same as accumulator  outputMin=[]  outputMax=[]  outputLastDataTypeStr=Inherit: Same as accumulator
  Freq1 : Constant  Value=2.4e6
  Mixer1 : Subsystem
  Real-Imag to Complex : RealImagToComplex
  Out1 : Outport
  wires:
  Constant/1 -> FIR Dec1/2
  Complex to Real-Imag/1 -> Mixer1/1(Input_I)
  Complex to Real-Imag1/1 -> Mixer1/3(DDS_I)
  Mixer1/2(Output_Q) -> Real-Imag to Complex/2
  Freq1/1 -> DDS_Gen1/1(In1)
  Complex to Real-Imag/2 -> Mixer1/2(Input_Q)
  Complex to Real-Imag1/2 -> Mixer1/4(DDS_Q)
  DDS_Gen1/1(Out1) -> Complex to Real-Imag1/1
  Real-Imag to Complex/1 -> FIR Dec1/1
  Mixer1/1(Output_I) -> Real-Imag to Complex/1
  FIR Dec1/1 -> Out1/1
  <IQ>/1 -> Complex to Real-Imag/1

== system Model/CORE_3_4/Path1 ==
  <IQ> : Inport
  Complex to Real-Imag : ComplexToRealImag
  Complex to Real-Imag1 : ComplexToRealImag
  Constant : Constant  Value=C12  SampleTime=dt0
  DDS_Gen1 : Subsystem
  FIR Dec1 : dspmlti4/FIR Decimation  FilterSource=Input port  h=designMultirateFIR(1,2)  D=2  filtStruct=Direct form  FilterObject=FDECIM  framing=Allow multirate processing  inputOffset=0  outputBufInitCond=0  roundingMode=Floor  overflowMode=off  firstCoeffDataTypeStr=Inherit: Same word length as input  firstCoeffMin=[]  firstCoeffMax=[]  firstCoeffLastDataTypeStr=Inherit: Same word length as input  outputDataTypeStr=Inherit: Same as accumulator  outputMin=[]  outputMax=[]  outputLastDataTypeStr=Inherit: Same as accumulator
  Freq1 : Constant  Value=2.4e6
  Mixer1 : Subsystem
  Real-Imag to Complex : RealImagToComplex
  Out1 : Outport
  wires:
  Constant/1 -> FIR Dec1/2
  Complex to Real-Imag/1 -> Mixer1/1(Input_I)
  Complex to Real-Imag1/1 -> Mixer1/3(DDS_I)
  Mixer1/2(Output_Q) -> Real-Imag to Complex/2
  Freq1/1 -> DDS_Gen1/1(In1)
  Complex to Real-Imag/2 -> Mixer1/2(Input_Q)
  Complex to Real-Imag1/2 -> Mixer1/4(DDS_Q)
  DDS_Gen1/1(Out1) -> Complex to Real-Imag1/1
  Real-Imag to Complex/1 -> FIR Dec1/1
  Mixer1/1(Output_I) -> Real-Imag to Complex/1
  FIR Dec1/1 -> Out1/1
  <IQ>/1 -> Complex to Real-Imag/1

== system Model/CORE_3_4/Path2 ==
  <IQ> : Inport
  Complex to Real-Imag : ComplexToRealImag
  Complex to Real-Imag1 : ComplexToRealImag
  Constant : Constant  Value=C12  SampleTime=dt0
  DDS_Gen1 : Subsystem
  FIR Dec1 : dspmlti4/FIR Decimation  FilterSource=Input port  h=designMultirateFIR(1,2)  D=2  filtStruct=Direct form  FilterObject=FDECIM  framing=Allow multirate processing  inputOffset=0  outputBufInitCond=0  roundingMode=Floor  overflowMode=off  firstCoeffDataTypeStr=Inherit: Same word length as input  firstCoeffMin=[]  firstCoeffMax=[]  firstCoeffLastDataTypeStr=Inherit: Same word length as input  outputDataTypeStr=Inherit: Same as accumulator  outputMin=[]  outputMax=[]  outputLastDataTypeStr=Inherit: Same as accumulator
  Freq1 : Constant  Value=2.4e6
  Mixer1 : Subsystem
  Real-Imag to Complex : RealImagToComplex
  Out1 : Outport
  wires:
  Constant/1 -> FIR Dec1/2
  Complex to Real-Imag/1 -> Mixer1/1(Input_I)
  Complex to Real-Imag1/1 -> Mixer1/3(DDS_I)
  Mixer1/2(Output_Q) -> Real-Imag to Complex/2
  Freq1/1 -> DDS_Gen1/1(In1)
  Complex to Real-Imag/2 -> Mixer1/2(Input_Q)
  Complex to Real-Imag1/2 -> Mixer1/4(DDS_Q)
  DDS_Gen1/1(Out1) -> Complex to Real-Imag1/1
  Real-Imag to Complex/1 -> FIR Dec1/1
  Mixer1/1(Output_I) -> Real-Imag to Complex/1
  FIR Dec1/1 -> Out1/1
  <IQ>/1 -> Complex to Real-Imag/1

== system Model/CORE_3_4/Path3 ==
  <IQ> : Inport
  Complex to Real-Imag : ComplexToRealImag
  Complex to Real-Imag1 : ComplexToRealImag
  Constant : Constant  Value=C12  SampleTime=dt0
  DDS_Gen1 : Subsystem
  FIR Dec1 : dspmlti4/FIR Decimation  FilterSource=Input port  h=designMultirateFIR(1,2)  D=2  filtStruct=Direct form  FilterObject=FDECIM  framing=Allow multirate processing  inputOffset=0  outputBufInitCond=0  roundingMode=Floor  overflowMode=off  firstCoeffDataTypeStr=Inherit: Same word length as input  firstCoeffMin=[]  firstCoeffMax=[]  firstCoeffLastDataTypeStr=Inherit: Same word length as input  outputDataTypeStr=Inherit: Same as accumulator  outputMin=[]  outputMax=[]  outputLastDataTypeStr=Inherit: Same as accumulator
  Freq1 : Constant  Value=2.4e6
  Mixer1 : Subsystem
  Real-Imag to Complex : RealImagToComplex
  Out1 : Outport
  wires:
  Constant/1 -> FIR Dec1/2
  Complex to Real-Imag/1 -> Mixer1/1(Input_I)
  Complex to Real-Imag1/1 -> Mixer1/3(DDS_I)
  Mixer1/2(Output_Q) -> Real-Imag to Complex/2
  Freq1/1 -> DDS_Gen1/1(In1)
  Complex to Real-Imag/2 -> Mixer1/2(Input_Q)
  Complex to Real-Imag1/2 -> Mixer1/4(DDS_Q)
  DDS_Gen1/1(Out1) -> Complex to Real-Imag1/1
  Real-Imag to Complex/1 -> FIR Dec1/1
  Mixer1/1(Output_I) -> Real-Imag to Complex/1
  FIR Dec1/1 -> Out1/1
  <IQ>/1 -> Complex to Real-Imag/1

== system Model/CORE_3_4/Path4 ==
  <IQ> : Inport
  Complex to Real-Imag : ComplexToRealImag
  Complex to Real-Imag1 : ComplexToRealImag
  Constant : Constant  Value=C12  SampleTime=dt0
  DDS_Gen1 : Subsystem
  FIR Dec1 : dspmlti4/FIR Decimation  FilterSource=Input port  h=designMultirateFIR(1,2)  D=2  filtStruct=Direct form  FilterObject=FDECIM  framing=Allow multirate processing  inputOffset=0  outputBufInitCond=0  roundingMode=Floor  overflowMode=off  firstCoeffDataTypeStr=Inherit: Same word length as input  firstCoeffMin=[]  firstCoeffMax=[]  firstCoeffLastDataTypeStr=Inherit: Same word length as input  outputDataTypeStr=Inherit: Same as accumulator  outputMin=[]  outputMax=[]  outputLastDataTypeStr=Inherit: Same as accumulator
  Freq1 : Constant  Value=2.4e6
  Mixer1 : Subsystem
  Real-Imag to Complex : RealImagToComplex
  Out1 : Outport
  wires:
  Constant/1 -> FIR Dec1/2
  Complex to Real-Imag/1 -> Mixer1/1(Input_I)
  Complex to Real-Imag1/1 -> Mixer1/3(DDS_I)
  Mixer1/2(Output_Q) -> Real-Imag to Complex/2
  Freq1/1 -> DDS_Gen1/1(In1)
  Complex to Real-Imag/2 -> Mixer1/2(Input_Q)
  Complex to Real-Imag1/2 -> Mixer1/4(DDS_Q)
  DDS_Gen1/1(Out1) -> Complex to Real-Imag1/1
  Real-Imag to Complex/1 -> FIR Dec1/1
  Mixer1/1(Output_I) -> Real-Imag to Complex/1
  FIR Dec1/1 -> Out1/1
  <IQ>/1 -> Complex to Real-Imag/1

== system Model/CORE_3_4/Path5 ==
  <IQ> : Inport
  Complex to Real-Imag : ComplexToRealImag
  Complex to Real-Imag1 : ComplexToRealImag
  Constant : Constant  Value=C12  SampleTime=dt0
  DDS_Gen1 : Subsystem
  FIR Dec1 : dspmlti4/FIR Decimation  FilterSource=Input port  h=designMultirateFIR(1,2)  D=2  filtStruct=Direct form  FilterObject=FDECIM  framing=Allow multirate processing  inputOffset=0  outputBufInitCond=0  roundingMode=Floor  overflowMode=off  firstCoeffDataTypeStr=Inherit: Same word length as input  firstCoeffMin=[]  firstCoeffMax=[]  firstCoeffLastDataTypeStr=Inherit: Same word length as input  outputDataTypeStr=Inherit: Same as accumulator  outputMin=[]  outputMax=[]  outputLastDataTypeStr=Inherit: Same as accumulator
  Freq1 : Constant  Value=2.4e6
  Mixer1 : Subsystem
  Real-Imag to Complex : RealImagToComplex
  Out1 : Outport
  wires:
  Constant/1 -> FIR Dec1/2
  Complex to Real-Imag/1 -> Mixer1/1(Input_I)
  Complex to Real-Imag1/1 -> Mixer1/3(DDS_I)
  Mixer1/2(Output_Q) -> Real-Imag to Complex/2
  Freq1/1 -> DDS_Gen1/1(In1)
  Complex to Real-Imag/2 -> Mixer1/2(Input_Q)
  Complex to Real-Imag1/2 -> Mixer1/4(DDS_Q)
  DDS_Gen1/1(Out1) -> Complex to Real-Imag1/1
  Real-Imag to Complex/1 -> FIR Dec1/1
  Mixer1/1(Output_I) -> Real-Imag to Complex/1
  FIR Dec1/1 -> Out1/1
  <IQ>/1 -> Complex to Real-Imag/1

== system Model/CORE_3_4/Path6 ==
  <IQ> : Inport
  Complex to Real-Imag : ComplexToRealImag
  Complex to Real-Imag1 : ComplexToRealImag
  Constant : Constant  Value=C12  SampleTime=dt0
  DDS_Gen1 : Subsystem
  FIR Dec1 : dspmlti4/FIR Decimation  FilterSource=Input port  h=designMultirateFIR(1,2)  D=2  filtStruct=Direct form  FilterObject=FDECIM  framing=Allow multirate processing  inputOffset=0  outputBufInitCond=0  roundingMode=Floor  overflowMode=off  firstCoeffDataTypeStr=Inherit: Same word length as input  firstCoeffMin=[]  firstCoeffMax=[]  firstCoeffLastDataTypeStr=Inherit: Same word length as input  outputDataTypeStr=Inherit: Same as accumulator  outputMin=[]  outputMax=[]  outputLastDataTypeStr=Inherit: Same as accumulator
  Freq1 : Constant  Value=2.4e6
  Mixer1 : Subsystem
  Real-Imag to Complex : RealImagToComplex
  Out1 : Outport
  wires:
  Constant/1 -> FIR Dec1/2
  Complex to Real-Imag/1 -> Mixer1/1(Input_I)
  Complex to Real-Imag1/1 -> Mixer1/3(DDS_I)
  Mixer1/2(Output_Q) -> Real-Imag to Complex/2
  Freq1/1 -> DDS_Gen1/1(In1)
  Complex to Real-Imag/2 -> Mixer1/2(Input_Q)
  Complex to Real-Imag1/2 -> Mixer1/4(DDS_Q)
  DDS_Gen1/1(Out1) -> Complex to Real-Imag1/1
  Real-Imag to Complex/1 -> FIR Dec1/1
  Mixer1/1(Output_I) -> Real-Imag to Complex/1
  FIR Dec1/1 -> Out1/1
  <IQ>/1 -> Complex to Real-Imag/1

== system Model/CORE_3_4/Path7 ==
  <IQ> : Inport
  Complex to Real-Imag : ComplexToRealImag
  Complex to Real-Imag1 : ComplexToRealImag
  Constant : Constant  Value=C12  SampleTime=dt0
  DDS_Gen1 : Subsystem
  FIR Dec1 : dspmlti4/FIR Decimation  FilterSource=Input port  h=designMultirateFIR(1,2)  D=2  filtStruct=Direct form  FilterObject=FDECIM  framing=Allow multirate processing  inputOffset=0  outputBufInitCond=0  roundingMode=Floor  overflowMode=off  firstCoeffDataTypeStr=Inherit: Same word length as input  firstCoeffMin=[]  firstCoeffMax=[]  firstCoeffLastDataTypeStr=Inherit: Same word length as input  outputDataTypeStr=Inherit: Same as accumulator  outputMin=[]  outputMax=[]  outputLastDataTypeStr=Inherit: Same as accumulator
  Freq1 : Constant  Value=2.4e6
  Mixer1 : Subsystem
  Real-Imag to Complex : RealImagToComplex
  Out1 : Outport
  wires:
  Constant/1 -> FIR Dec1/2
  Complex to Real-Imag/1 -> Mixer1/1(Input_I)
  Complex to Real-Imag1/1 -> Mixer1/3(DDS_I)
  Mixer1/2(Output_Q) -> Real-Imag to Complex/2
  Freq1/1 -> DDS_Gen1/1(In1)
  Complex to Real-Imag/2 -> Mixer1/2(Input_Q)
  Complex to Real-Imag1/2 -> Mixer1/4(DDS_Q)
  DDS_Gen1/1(Out1) -> Complex to Real-Imag1/1
  Real-Imag to Complex/1 -> FIR Dec1/1
  Mixer1/1(Output_I) -> Real-Imag to Complex/1
  FIR Dec1/1 -> Out1/1
  <IQ>/1 -> Complex to Real-Imag/1

== system Model/CORE_3_4/Path8 ==
  <IQ> : Inport
  Complex to Real-Imag : ComplexToRealImag
  Complex to Real-Imag1 : ComplexToRealImag
  Constant : Constant  Value=C12  SampleTime=dt0
  DDS_Gen1 : Subsystem
  FIR Dec1 : dspmlti4/FIR Decimation  FilterSource=Input port  h=designMultirateFIR(1,2)  D=2  filtStruct=Direct form  FilterObject=FDECIM  framing=Allow multirate processing  inputOffset=0  outputBufInitCond=0  roundingMode=Floor  overflowMode=off  firstCoeffDataTypeStr=Inherit: Same word length as input  firstCoeffMin=[]  firstCoeffMax=[]  firstCoeffLastDataTypeStr=Inherit: Same word length as input  outputDataTypeStr=Inherit: Same as accumulator  outputMin=[]  outputMax=[]  outputLastDataTypeStr=Inherit: Same as accumulator
  Freq1 : Constant  Value=2.4e6
  Mixer1 : Subsystem
  Real-Imag to Complex : RealImagToComplex
  Out1 : Outport
  wires:
  Constant/1 -> FIR Dec1/2
  Complex to Real-Imag/1 -> Mixer1/1(Input_I)
  Complex to Real-Imag1/1 -> Mixer1/3(DDS_I)
  Mixer1/2(Output_Q) -> Real-Imag to Complex/2
  Freq1/1 -> DDS_Gen1/1(In1)
  Complex to Real-Imag/2 -> Mixer1/2(Input_Q)
  Complex to Real-Imag1/2 -> Mixer1/4(DDS_Q)
  DDS_Gen1/1(Out1) -> Complex to Real-Imag1/1
  Real-Imag to Complex/1 -> FIR Dec1/1
  Mixer1/1(Output_I) -> Real-Imag to Complex/1
  FIR Dec1/1 -> Out1/1
  <IQ>/1 -> Complex to Real-Imag/1

== system Model/CORE_3_5/Path1 ==
  <IQ> : Inport
  Complex to Real-Imag : ComplexToRealImag
  Complex to Real-Imag1 : ComplexToRealImag
  Constant : Constant  Value=C12  SampleTime=dt0
  DDS_Gen1 : Subsystem
  FIR Dec1 : dspmlti4/FIR Decimation  FilterSource=Input port  h=designMultirateFIR(1,2)  D=2  filtStruct=Direct form  FilterObject=FDECIM  framing=Allow multirate processing  inputOffset=0  outputBufInitCond=0  roundingMode=Floor  overflowMode=off  firstCoeffDataTypeStr=Inherit: Same word length as input  firstCoeffMin=[]  firstCoeffMax=[]  firstCoeffLastDataTypeStr=Inherit: Same word length as input  outputDataTypeStr=Inherit: Same as accumulator  outputMin=[]  outputMax=[]  outputLastDataTypeStr=Inherit: Same as accumulator
  Freq1 : Constant  Value=2.4e6
  Mixer1 : Subsystem
  Real-Imag to Complex : RealImagToComplex
  Out1 : Outport
  wires:
  Constant/1 -> FIR Dec1/2
  Complex to Real-Imag/1 -> Mixer1/1(Input_I)
  Complex to Real-Imag1/1 -> Mixer1/3(DDS_I)
  Mixer1/2(Output_Q) -> Real-Imag to Complex/2
  Freq1/1 -> DDS_Gen1/1(In1)
  Complex to Real-Imag/2 -> Mixer1/2(Input_Q)
  Complex to Real-Imag1/2 -> Mixer1/4(DDS_Q)
  DDS_Gen1/1(Out1) -> Complex to Real-Imag1/1
  Real-Imag to Complex/1 -> FIR Dec1/1
  Mixer1/1(Output_I) -> Real-Imag to Complex/1
  FIR Dec1/1 -> Out1/1
  <IQ>/1 -> Complex to Real-Imag/1

== system Model/CORE_3_5/Path2 ==
  <IQ> : Inport
  Complex to Real-Imag : ComplexToRealImag
  Complex to Real-Imag1 : ComplexToRealImag
  Constant : Constant  Value=C12  SampleTime=dt0
  DDS_Gen1 : Subsystem
  FIR Dec1 : dspmlti4/FIR Decimation  FilterSource=Input port  h=designMultirateFIR(1,2)  D=2  filtStruct=Direct form  FilterObject=FDECIM  framing=Allow multirate processing  inputOffset=0  outputBufInitCond=0  roundingMode=Floor  overflowMode=off  firstCoeffDataTypeStr=Inherit: Same word length as input  firstCoeffMin=[]  firstCoeffMax=[]  firstCoeffLastDataTypeStr=Inherit: Same word length as input  outputDataTypeStr=Inherit: Same as accumulator  outputMin=[]  outputMax=[]  outputLastDataTypeStr=Inherit: Same as accumulator
  Freq1 : Constant  Value=2.4e6
  Mixer1 : Subsystem
  Real-Imag to Complex : RealImagToComplex
  Out1 : Outport
  wires:
  Constant/1 -> FIR Dec1/2
  Complex to Real-Imag/1 -> Mixer1/1(Input_I)
  Complex to Real-Imag1/1 -> Mixer1/3(DDS_I)
  Mixer1/2(Output_Q) -> Real-Imag to Complex/2
  Freq1/1 -> DDS_Gen1/1(In1)
  Complex to Real-Imag/2 -> Mixer1/2(Input_Q)
  Complex to Real-Imag1/2 -> Mixer1/4(DDS_Q)
  DDS_Gen1/1(Out1) -> Complex to Real-Imag1/1
  Real-Imag to Complex/1 -> FIR Dec1/1
  Mixer1/1(Output_I) -> Real-Imag to Complex/1
  FIR Dec1/1 -> Out1/1
  <IQ>/1 -> Complex to Real-Imag/1

== system Model/CORE_3_5/Path3 ==
  <IQ> : Inport
  Complex to Real-Imag : ComplexToRealImag
  Complex to Real-Imag1 : ComplexToRealImag
  Constant : Constant  Value=C12  SampleTime=dt0
  DDS_Gen1 : Subsystem
  FIR Dec1 : dspmlti4/FIR Decimation  FilterSource=Input port  h=designMultirateFIR(1,2)  D=2  filtStruct=Direct form  FilterObject=FDECIM  framing=Allow multirate processing  inputOffset=0  outputBufInitCond=0  roundingMode=Floor  overflowMode=off  firstCoeffDataTypeStr=Inherit: Same word length as input  firstCoeffMin=[]  firstCoeffMax=[]  firstCoeffLastDataTypeStr=Inherit: Same word length as input  outputDataTypeStr=Inherit: Same as accumulator  outputMin=[]  outputMax=[]  outputLastDataTypeStr=Inherit: Same as accumulator
  Freq1 : Constant  Value=2.4e6
  Mixer1 : Subsystem
  Real-Imag to Complex : RealImagToComplex
  Out1 : Outport
  wires:
  Constant/1 -> FIR Dec1/2
  Complex to Real-Imag/1 -> Mixer1/1(Input_I)
  Complex to Real-Imag1/1 -> Mixer1/3(DDS_I)
  Mixer1/2(Output_Q) -> Real-Imag to Complex/2
  Freq1/1 -> DDS_Gen1/1(In1)
  Complex to Real-Imag/2 -> Mixer1/2(Input_Q)
  Complex to Real-Imag1/2 -> Mixer1/4(DDS_Q)
  DDS_Gen1/1(Out1) -> Complex to Real-Imag1/1
  Real-Imag to Complex/1 -> FIR Dec1/1
  Mixer1/1(Output_I) -> Real-Imag to Complex/1
  FIR Dec1/1 -> Out1/1
  <IQ>/1 -> Complex to Real-Imag/1

== system Model/CORE_3_5/Path4 ==
  <IQ> : Inport
  Complex to Real-Imag : ComplexToRealImag
  Complex to Real-Imag1 : ComplexToRealImag
  Constant : Constant  Value=C12  SampleTime=dt0
  DDS_Gen1 : Subsystem
  FIR Dec1 : dspmlti4/FIR Decimation  FilterSource=Input port  h=designMultirateFIR(1,2)  D=2  filtStruct=Direct form  FilterObject=FDECIM  framing=Allow multirate processing  inputOffset=0  outputBufInitCond=0  roundingMode=Floor  overflowMode=off  firstCoeffDataTypeStr=Inherit: Same word length as input  firstCoeffMin=[]  firstCoeffMax=[]  firstCoeffLastDataTypeStr=Inherit: Same word length as input  outputDataTypeStr=Inherit: Same as accumulator  outputMin=[]  outputMax=[]  outputLastDataTypeStr=Inherit: Same as accumulator
  Freq1 : Constant  Value=2.4e6
  Mixer1 : Subsystem
  Real-Imag to Complex : RealImagToComplex
  Out1 : Outport
  wires:
  Constant/1 -> FIR Dec1/2
  Complex to Real-Imag/1 -> Mixer1/1(Input_I)
  Complex to Real-Imag1/1 -> Mixer1/3(DDS_I)
  Mixer1/2(Output_Q) -> Real-Imag to Complex/2
  Freq1/1 -> DDS_Gen1/1(In1)
  Complex to Real-Imag/2 -> Mixer1/2(Input_Q)
  Complex to Real-Imag1/2 -> Mixer1/4(DDS_Q)
  DDS_Gen1/1(Out1) -> Complex to Real-Imag1/1
  Real-Imag to Complex/1 -> FIR Dec1/1
  Mixer1/1(Output_I) -> Real-Imag to Complex/1
  FIR Dec1/1 -> Out1/1
  <IQ>/1 -> Complex to Real-Imag/1
